simulink model "EulerEqs_axisymmetric_analytical"  (R2020b)
settings: Solver=FixedStepAuto  StartTime=0.0  StopTime=10.0  FixedStep=sim_constants.time_step  RelTol=1e-3
undefined symbols (not defined in the file or in its folder): i, sim_constants
settings Model: Creator=valerie  LastModifiedBy=valerie

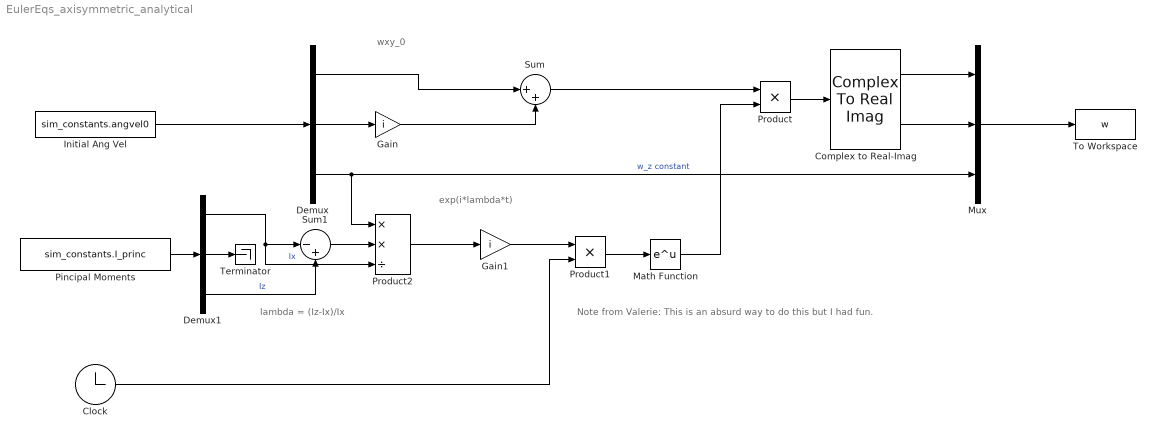
== system EulerEqs_axisymmetric_analytical ==
  note: exp(i*lambda*t)
  note: lambda = (Iz-Ix)/Ix
  note: wxy_0
  note: Note from Valerie: This is an absurd way to do this but I had fun.
  Clock : Clock
      settings: Decimation=sim_constants.time_step
  Complex to Real-Imag : ComplexToRealImag
  Demux : Demux  Outputs=3
  Demux1 : Demux  Outputs=3
  Gain : Gain  Gain=i
  Gain1 : Gain  Gain=i
  Initial Ang Vel : Constant  Value=sim_constants.angvel0
  Math Function : Math  SaturateOnIntegerOverflow=on
  Mux : Mux  Inputs=3
  Pincipal Moments : Constant  Value=sim_constants.I_princ
  Product : Product
  Product1 : Product
  Product2 : Product  Inputs=**/
  Sum : Sum  Inputs=|++
  Sum1 : Sum  Inputs=|-+
  Terminator : Terminator
  To Workspace : ToWorkspace  VariableName=w  SampleTime=-1
  wires:
  Initial Ang Vel/1 -> Demux/1
  Demux/3 -> Product2/1, Mux/3  "w_z constant"
  Pincipal Moments/1 -> Demux1/1
  Demux/1 -> Sum/1
  Demux/2 -> Gain/1
  Gain/1 -> Sum/2
  Mux/1 -> To Workspace/1
  Product2/1 -> Gain1/1
  Gain1/1 -> Product1/1
  Clock/1 -> Product1/2
  Sum/1 -> Product/1
  Complex to Real-Imag/1 -> Mux/1
  Complex to Real-Imag/2 -> Mux/2
  Product1/1 -> Math Function/1
  Math Function/1 -> Product/2
  Product/1 -> Complex to Real-Imag/1
  Demux1/2 -> Terminator/1
  Demux1/1 -> Product2/3, Sum1/1  "Ix"
  Demux1/3 -> Sum1/2  "Iz"
  Sum1/1 -> Product2/2
